simulink library "Lib_Turbo_Shaft_TMATS"  (R2019b)
settings: Solver=ode45  StartTime=0.0  StopTime=10.0  RelTol=1e-3  EnableMultiTasking=on
Description:
  | Thomas Modules
settings Model: Creator=jwchapm2  LastModifiedBy=bhisma
settings DataIOCC: LimitDataPoints=on  SaveFormat=Array  ReturnWorkspaceOutputs=off
settings OptimizationCC: ExpressionDepthLimit=2147483647  LifeSpan=inf
settings DebuggingCC: UnderspecifiedInitializationDetection=Classic  MergeDetectMultiDrivingBlocksExec=none  SolverPrmCheckMsg=warning  StateNameClashWarn=warning  SFUnexpectedBacktrackingDiag=warning  SFNoUnconditionalDefaultTransitionDiag=warning  SFExecutionAtInitializationDiag=none  ArithmeticOperatorsInVariantConditions=warning
settings HardwareCC: ProdBitPerPointer=32  ProdBitPerSizeT=32  ProdBitPerPtrDiffT=32  ProdLargestAtomicFloat=None  ProdIntDivRoundTo=Undefined  ProdEndianess=Unspecified  ProdWordSize=32  ProdHWDeviceType=32-bit Generic
settings ModelReferenceCC: PropagateSignalLabelsOutOfModel=off
settings SFSimCC: SimUseLocalCustomCode=off  CustomCodeUndefinedFunction=UseInterfaceOnly
settings RTWCC: RTWUseLocalCustomCode=off
settings CodeAppCC: StateflowObjectComments=on
settings GRTTargetCC: TargetLangStandard=C89/C90 (ANSI)  GeneratePreprocessorConditionals=Disable all
settings ConfigComp: CovMetricSettings=dw  CovHtmlReporting=on  CovSaveCumulativeToWorkspaceVar=on  CovSaveSingleToWorkspaceVar=on  CovExternalEMLEnable=off

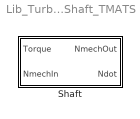
== system Lib_Turbo_Shaft_TMATS ==
  Shaft : Subsystem  mask(T-MATS: Shaft Library Block){Shaft_Inertia_M=0.3183}
      mask prompts: Shaft_Inertia_M "Shaft_Inertia_M - Shaft Inertia Term [slugs*ft2]"
      mask help: This block simulates the performance of a shaft using basic dynamic equations and properties.
      mask Help: web(which('Turbo_TMATS_Shft.html'),'-helpbrowser')

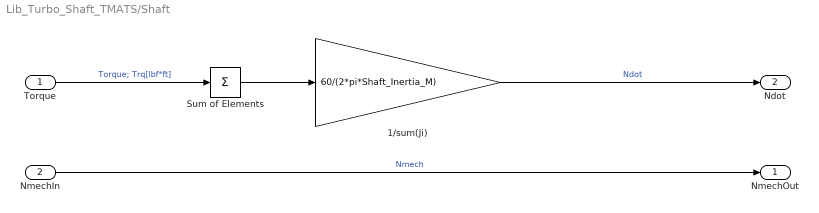
== system Lib_Turbo_Shaft_TMATS/Shaft ==
  Torque : Inport
  NmechIn : Inport  Port=2
  1/sum(Ji) : Gain  Gain=60/(2*pi*Shaft_Inertia_M)  SaturateOnIntegerOverflow=on  OutDataTypeStr=Inherit: Same as input  ParamDataTypeStr=Inherit: Same as input
  Sum of Elements : Sum  Inputs=+
  NmechOut : Outport
  Ndot : Outport  Port=2
  wires:
  NmechIn/1 -> NmechOut/1  "Nmech"
  1/sum(Ji)/1 -> Ndot/1  "Ndot"
  Torque/1 -> Sum of Elements/1  "Torque; Trq[lbf*ft]"
  Sum of Elements/1 -> 1/sum(Ji)/1
